simulink model "Representacion_Estado_Discretos1"  (R2017a)
settings: Solver=VariableStepAuto  StartTime=0.0  StopTime=60  RelTol=1e-3
values from neighbouring files (symbols this model uses):
  Ad = [0 1;-a2 -a1]    [Representacion_Estado_Discretos.m]
  Bd = [0;b]    [Representacion_Estado_Discretos.m]
  Cd = [1,0]    [Representacion_Estado_Discretos.m]
settings Model: Creator=franj  LastModifiedBy=franj

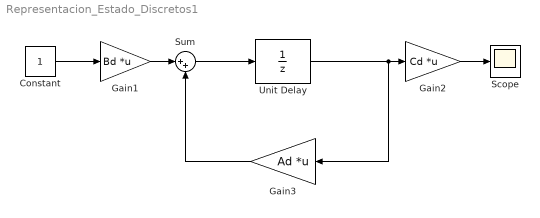
== system Representacion_Estado_Discretos1 ==
  Constant : Constant
  Gain1 : Gain  Gain=Bd  Multiplication=Matrix(K*u)
  Gain2 : Gain  Gain=Cd  Multiplication=Matrix(K*u)
  Gain3 : Gain  Gain=Ad  Multiplication=Matrix(K*u)
  Scope : Scope
  Sum : Sum  Inputs=|++
  Unit Delay : UnitDelay
  wires:
  Constant/1 -> Gain1/1
  Gain1/1 -> Sum/1
  Sum/1 -> Unit Delay/1
  Gain2/1 -> Scope/1
  Unit Delay/1 -> Gain3/1, Gain2/1
  Gain3/1 -> Sum/2
